simulink model "Target_Control_System"  (R2021b)
settings: Solver=FixedStepDiscrete  StartTime=0.0  StopTime=5  RelTol=1e-3
PreLoadFcn:
  | RTWConfigurationCB('preloadfcn', bdroot);
PostLoadFcn:
  | load('configuration/data_struct.mat');
  | load('configuration/fluxMaps_propMotor.mat');
  | load('configuration/parameterInit_PROP.mat');
  | load('configuration/parameterInit_PUMP.mat');
  | load('configuration/parameterInit_PITCH.mat');
  | load('configuration/parameterInit_TILT.mat');
  | %load('configuration/base_workspace_signal_definition.mat');
  | %load('resolvedatastores_to_baseworkspace_for_faster_simulation.mat');
model workspace (MAT data in the model file):
  SIMULATION_OPTIONS : Simulink.Parameter (value not decoded)
  TARGET_CODE_GEN : Simulink.Parameter (value not decoded)
  TCS_SAMPLE_FREQ_HZ : Simulink.Parameter (value not decoded)
symbols that are objects in the model workspace (value not decoded): TARGET_CODE_GEN, TCS_SAMPLE_FREQ_HZ
undefined symbols (not defined in the file): A_DQ_REF_LPF_INIT__PITCH, A_DQ_REF_LPF_INIT__PROP, A_DQ_REF_LPF_INIT__PUMP, A_DQ_REF_LPF_INIT__TILT, A_OBSERVER_CONFIDENCE_INIT__PITCH, A_OBSERVER_CONFIDENCE_INIT__PROP, A_OBSERVER_CONFIDENCE_INIT__PUMP, A_OBSERVER_CONFIDENCE_INIT__TILT, ACTUATOR_MAX_ANGLE_TRIP__PITCH, ACTUATOR_MIN_ANGLE_TRIP__PITCH, ACTUATOR_POS_SENSOR_INV_DIRECTION__PITCH, ACTUATOR_POS_SENSOR_INV_DIRECTION__TILT, ACTUATOR_POS_SENSOR_OFFSET__PITCH, ACTUATOR_POS_SENSOR_OFFSET__TILT, ADC_scaler1_baseaddr_TILT, ADC_SCALER_FLOAT_TO_FIXPOINT_EXPANSION, ANGLE_ELEC_FROM_SENSOR_OFFSET_INIT__PITCH, ANGLE_ELEC_FROM_SENSOR_OFFSET_INIT__PROP, ANGLE_ELEC_FROM_SENSOR_OFFSET_INIT__PUMP, ANGLE_ELEC_FROM_SENSOR_OFFSET_INIT__TILT, AUTO_CLEAR_FAULTS_ENABLED__PITCH, AUTO_CLEAR_FAULTS_ENABLED__PROP, AUTO_CLEAR_FAULTS_ENABLED__PUMP, AUTO_CLEAR_FAULTS_ENABLED__TILT, AUTO_CLEAR_FAULTS_WAIT_TICKS__PITCH, AUTO_CLEAR_FAULTS_WAIT_TICKS__PROP, AUTO_CLEAR_FAULTS_WAIT_TICKS__PUMP, AUTO_CLEAR_FAULTS_WAIT_TICKS__TILT, AUTO_I_ZERO_IDLE_TICKS__PITCH, AUTO_I_ZERO_IDLE_TICKS__PROP, AUTO_I_ZERO_IDLE_TICKS__PUMP, AUTO_I_ZERO_IDLE_TICKS__TILT, AUTO_I_ZERO_OFFSET_IDC_THRESHOLD__PITCH, AUTO_I_ZERO_OFFSET_IDC_THRESHOLD__PROP, AUTO_I_ZERO_OFFSET_IDC_THRESHOLD__PUMP, AUTO_I_ZERO_OFFSET_IDC_THRESHOLD__TILT, AUTO_I_ZERO_OFFSET_IPH_THRESHOLD__PITCH, AUTO_I_ZERO_OFFSET_IPH_THRESHOLD__PROP, AUTO_I_ZERO_OFFSET_IPH_THRESHOLD__PUMP, AUTO_I_ZERO_OFFSET_IPH_THRESHOLD__TILT, AUTO_SENSORLESS_SWITCHOVER_DISABLE_OMEGA, AUTO_SENSORLESS_SWITCHOVER_ENABLE_OMEGA, AUTO_SENSORLESS_SWITCHOVER_MIN_CONFIDENCE, AUXILIARY_PROTECTION_UNIT_BASEADDR__TILT, blanking_max_error_omega_INIT_PITCH, blanking_max_error_omega_INIT_TILT, blanking_max_error_position_INIT_PITCH, blanking_max_error_position_INIT_TILT, BRUTE_START_I_Q_REF_RAMP_SPEED__PITCH, BRUTE_START_I_Q_REF_RAMP_SPEED__PROP, BRUTE_START_I_Q_REF_RAMP_SPEED__PUMP, BRUTE_START_I_Q_REF_RAMP_SPEED__TILT, CONTROL_LOOP_DT_INIT__PITCH, CONTROL_LOOP_DT_INIT__PROP, CONTROL_LOOP_DT_INIT__PUMP, CONTROL_LOOP_DT_INIT__TILT, CORRECTION_FILTER_SCALE__PITCH, CORRECTION_FILTER_SCALE__PROP, CORRECTION_FILTER_SCALE__PUMP, CORRECTION_FILTER_SCALE__TILT ... (+458)
libraries: simulink x178, Reusables_Lib x24
(part 20 of 47)

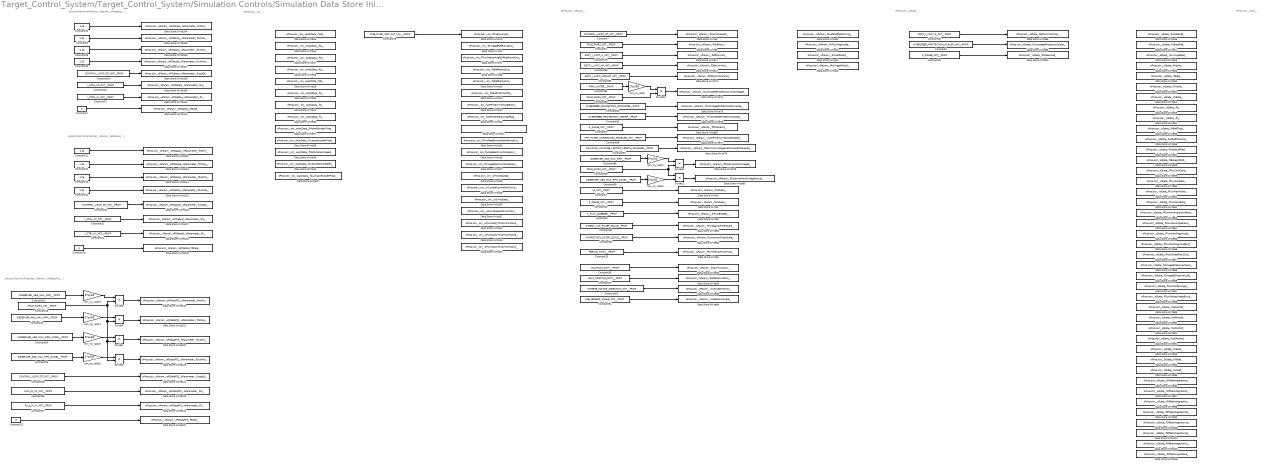
== system Target_Control_System/Target_Control_System/Simulation Controls/Simulation Data Store Initialization/parameter_init_prop/initializeIntTaskParametersPropulsion() ==
  note: oProp.oIsr_.oOut_...
  note: piControllerInit(oProp.oIsr_.oParam_.oPiDataPll2_...)
  note: piControllerInit(oProp.oIsr_.oParam_.oPiDataId_...)
  note: piControllerInit(oProp.oIsr_.oParam_.oPiDataIq_...)
  note: oProp.oIsr_.oState_...
  note: oProp.oIsr_.oIn_...
  note: oProp.oIsr_.oParam_...
  Constant1 : Constant  Value=0  OutDataTypeStr=single  SampleTime=-1
  Constant{10..11,13,29} (4 alike) : Constant  Value=-1.15  OutDataTypeStr=single  SampleTime=-1
  Constant{8,12,14,30} (4 alike) : Constant  Value=1.15  OutDataTypeStr=single  SampleTime=-1
  Constant15 : Constant  Value=0  OutDataTypeStr=single  SampleTime=-1
  Constant18 : Constant  Value=-OBSERVER_ABS_MAX_RPM__PROP  OutDataTypeStr=single  SampleTime=-1
  Constant{3,19,83,90} (4 alike) : Constant  Value=POLE_PAIRS_INIT__PROP  OutDataTypeStr=single  SampleTime=-1
  Constant2 : Constant  Value=LS_INIT__PROP  OutDataTypeStr=single  SampleTime=-1
  Constant20 : Constant  Value=OBSERVER_ABS_MAX_RPM__PROP  OutDataTypeStr=single  SampleTime=-1
  Constant21 : Constant  Value=I_CTRL_KI_INIT__PROP  OutDataTypeStr=single  SampleTime=-1
  Constant22 : Constant  Value=I_CTRL_KI_INIT__PROP  OutDataTypeStr=single  SampleTime=-1
  Constant23 : Constant  Value=0  OutDataTypeStr=single  SampleTime=-1
  Constant24 : Constant  Value=-OBSERVER_ABS_MAX_RPM_ACCEL__PROP  OutDataTypeStr=single  SampleTime=-1
  Constant25 : Constant  Value=PERIOD_TICKS__PROP  OutDataTypeStr=single  SampleTime=-1
  Constant26 : Constant  Value=OBSERVER_ABS_MAX_RPM_ACCEL__PROP  OutDataTypeStr=single  SampleTime=-1
  Constant27 : Constant  Value=PLL2_PI_KI_INIT__PROP  OutDataTypeStr=single  SampleTime=-1
  Constant{7,28,31,33} (4 alike) : Constant  Value=CONTROL_LOOP_DT_INIT__PROP  OutDataTypeStr=single  SampleTime=-1
  Constant32 : Constant  Value=I_CTRL_KP_INIT__PROP  OutDataTypeStr=single  SampleTime=-1
  Constant34 : Constant  Value=I_CTRL_KP_INIT__PROP  OutDataTypeStr=single  SampleTime=-1
  Constant35 : Constant  Value=PLL2_PI_KP_INIT__PROP  OutDataTypeStr=single  SampleTime=-1
  Constant37 : Constant  Value=HALF_POSITIVE_DUTY__PROP  OutDataTypeStr=single  SampleTime=-1
  Constant38 : Constant  Value=MAXIMUM_DUTY__PROP  OutDataTypeStr=single  SampleTime=-1
  Constant39 : Constant  Value=R_PHASE_INIT__PROP  OutDataTypeStr=single  SampleTime=-1
  Constant40 : Constant  Value=R_PHASE_INIT__PROP  OutDataTypeStr=single  SampleTime=-1
  Constant5 : Constant  Value=OVERSPEED_PROTECTION_SCALER_INIT__PROP  OutDataTypeStr=single  SampleTime=-1
  Constant6 : Constant  Value=R_PHASE_INIT__PROP  OutDataTypeStr=single  SampleTime=-1
  Constant78 : Constant  Value=ONE_OVER_UDC_INIT_VAL__PROP  OutDataTypeStr=single  SampleTime=-1
  Constant79 : Constant  Value=SOFT_I_LIMIT_A_INIT__PROP  OutDataTypeStr=single  SampleTime=-1
  Constant80 : Constant  Value=SOFT_I_LIMIT_KP_INIT__PROP  OutDataTypeStr=single  SampleTime=-1
  Constant81 : Constant  Value=SOFT_I_LIMIT_UPRAMP_INIT__PROP  OutDataTypeStr=single  SampleTime=-1
  Constant82 : Constant  Value=RPM_LIMITER__PROP  OutDataTypeStr=single  SampleTime=-1
  Constant84 : Constant  Value=OVERSPEED_PROTECTION_DOWNSTEP__PROP  OutDataTypeStr=single  SampleTime=-1
  Constant85 : Constant  Value=OVERSPEED_PROTECTION_UPSTEP__PROP  OutDataTypeStr=single  SampleTime=-1
  Constant86 : Constant  Value=UPH_FILTER_CORRECTION_ENABLED_INIT__PROP  OutDataTypeStr=uint32  SampleTime=-1
  Constant87 : Constant  Value=MAXIMUM_VOLTAGE_VECTOR_LENGTH_SQUARED__PROP  OutDataTypeStr=single  SampleTime=-1
  Constant88 : Constant  Value=OBSERVER_ABS_MAX_RPM__PROP  OutDataTypeStr=single  SampleTime=-1
  Constant89 : Constant  Value=OBSERVER_ABS_MAX_RPM_ACCEL__PROP  OutDataTypeStr=single  SampleTime=-1
  Constant9 : Constant  Value=K_FLUX_BLEEDER__PROP  OutDataTypeStr=single  SampleTime=-1
  Constant91 : Constant  Value=OMEGA_VAR_FILTER_SCALE__PROP  OutDataTypeStr=single  SampleTime=-1
  Constant92 : Constant  Value=CORRECTION_FILTER_SCALE__PROP  OutDataTypeStr=single  SampleTime=-1
  Constant93 : Constant  Value=INVERSE_MOTOR_DIRECTION_INIT__PROP  OutDataTypeStr=int32  SampleTime=-1
  Constant94 : Constant  Value=USE_SENSOR_ANGLE_INIT__PROP  OutDataTypeStr=int32  SampleTime=-1
  Constant95 : Constant  Value=SOFT_I_LIMIT_A_INIT__PROP  OutDataTypeStr=single  SampleTime=-1
  Data Store Write1 : DataStoreWrite  DataStoreName=oProp  DataStoreElements=oProp.oIsr_.oIn_.fOmegaERefRampOut_  IndexOptions=Index vector (dialog)  Indices=1  OutputSizes=1
  Data Store Write10 : DataStoreWrite  DataStoreName=oProp  DataStoreElements=oProp.oIsr_.oIn_.fIdRefRampOut_  IndexOptions=Index vector (dialog)  Indices=1  OutputSizes=1
  Data Store Write100 : DataStoreWrite  DataStoreName=oProp  DataStoreElements=oProp.oIsr_.oState_.fOffsetIntegratorUa_  IndexOptions=Index vector (dialog)  Indices=1  OutputSizes=1
  Data Store Write101 : DataStoreWrite  DataStoreName=oProp  DataStoreElements=oProp.oIsr_.oState_.fOffsetIntegratorUb_  IndexOptions=Index vector (dialog)  Indices=1  OutputSizes=1
  Data Store Write102 : DataStoreWrite  DataStoreName=oProp  DataStoreElements=oProp.oIsr_.oState_.fOffsetIntegratorUc_  IndexOptions=Index vector (dialog)  Indices=1  OutputSizes=1
  Data Store Write103 : DataStoreWrite  DataStoreName=oProp  DataStoreElements=oProp.oIsr_.oState_.fOffsetAvgUphase_  IndexOptions=Index vector (dialog)  Indices=1  OutputSizes=1
  Data Store Write104 : DataStoreWrite  DataStoreName=oProp  DataStoreElements=oProp.oIsr_.oParam_.oPiDataIq_.oParameter_.fIntMin_  IndexOptions=Index vector (dialog)  Indices=1  OutputSizes=1
  Data Store Write105 : DataStoreWrite  DataStoreName=oProp  DataStoreElements=oProp.oIsr_.oParam_.oPiDataIq_.oParameter_.fIntMax_  IndexOptions=Index vector (dialog)  Indices=1  OutputSizes=1
  Data Store Write106 : DataStoreWrite  DataStoreName=oProp  DataStoreElements=oProp.oIsr_.oParam_.oPiDataIq_.oParameter_.fOutMin_  IndexOptions=Index vector (dialog)  Indices=1  OutputSizes=1
  Data Store Write107 : DataStoreWrite  DataStoreName=oProp  DataStoreElements=oProp.oIsr_.oParam_.oPiDataIq_.oParameter_.fOutMax_  IndexOptions=Index vector (dialog)  Indices=1  OutputSizes=1
  Data Store Write108 : DataStoreWrite  DataStoreName=oProp  DataStoreElements=oProp.oIsr_.oParam_.oPiDataIq_.oParameter_.fLoopDt_  IndexOptions=Index vector (dialog)  Indices=1  OutputSizes=1
  Data Store Write109 : DataStoreWrite  DataStoreName=oProp  DataStoreElements=oProp.oIsr_.oParam_.oPiDataIq_.oParameter_.fKp_  IndexOptions=Index vector (dialog)  Indices=1  OutputSizes=1
  Data Store Write11 : DataStoreWrite  DataStoreName=oProp  DataStoreElements=oProp.oIsr_.oIn_.fIdRefFractionOfIq_  IndexOptions=Index vector (dialog)  Indices=1  OutputSizes=1
  Data Store Write110 : DataStoreWrite  DataStoreName=oProp  DataStoreElements=oProp.oIsr_.oParam_.oPiDataIq_.oParameter_.fKi_  IndexOptions=Index vector (dialog)  Indices=1  OutputSizes=1
  Data Store Write111 : DataStoreWrite  DataStoreName=oProp  DataStoreElements=oProp.oIsr_.oParam_.oPiDataIq_.fState_  IndexOptions=Index vector (dialog)  Indices=1  OutputSizes=1
  Data Store Write112 : DataStoreWrite  DataStoreName=oProp  DataStoreElements=oProp.oIsr_.oParam_.oPiDataId_.oParameter_.fIntMin_  IndexOptions=Index vector (dialog)  Indices=1  OutputSizes=1
  Data Store Write113 : DataStoreWrite  DataStoreName=oProp  DataStoreElements=oProp.oIsr_.oParam_.oPiDataId_.oParameter_.fIntMax_  IndexOptions=Index vector (dialog)  Indices=1  OutputSizes=1
  Data Store Write114 : DataStoreWrite  DataStoreName=oProp  DataStoreElements=oProp.oIsr_.oParam_.oPiDataId_.oParameter_.fOutMin_  IndexOptions=Index vector (dialog)  Indices=1  OutputSizes=1
  Data Store Write115 : DataStoreWrite  DataStoreName=oProp  DataStoreElements=oProp.oIsr_.oParam_.oPiDataId_.oParameter_.fOutMax_  IndexOptions=Index vector (dialog)  Indices=1  OutputSizes=1
  Data Store Write116 : DataStoreWrite  DataStoreName=oProp  DataStoreElements=oProp.oIsr_.oParam_.oPiDataId_.oParameter_.fLoopDt_  IndexOptions=Index vector (dialog)  Indices=1  OutputSizes=1
  Data Store Write117 : DataStoreWrite  DataStoreName=oProp  DataStoreElements=oProp.oIsr_.oParam_.oPiDataId_.oParameter_.fKp_  IndexOptions=Index vector (dialog)  Indices=1  OutputSizes=1
  Data Store Write118 : DataStoreWrite  DataStoreName=oProp  DataStoreElements=oProp.oIsr_.oParam_.oPiDataId_.oParameter_.fKi_  IndexOptions=Index vector (dialog)  Indices=1  OutputSizes=1
  Data Store Write119 : DataStoreWrite  DataStoreName=oProp  DataStoreElements=oProp.oIsr_.oParam_.oPiDataId_.fState_  IndexOptions=Index vector (dialog)  Indices=1  OutputSizes=1
  Data Store Write12 : DataStoreWrite  DataStoreName=oProp  DataStoreElements=oProp.oIsr_.oIn_.fUphFilterAmplitudeRatio_  IndexOptions=Index vector (dialog)  Indices=1  OutputSizes=1
  Data Store Write120 : DataStoreWrite  DataStoreName=oProp  DataStoreElements=oProp.oIsr_.oParam_.oPiDataPll2_.oParameter_.fIntMin_  IndexOptions=Index vector (dialog)  Indices=1  OutputSizes=1
  Data Store Write121 : DataStoreWrite  DataStoreName=oProp  DataStoreElements=oProp.oIsr_.oParam_.oPiDataPll2_.oParameter_.fIntMax_  IndexOptions=Index vector (dialog)  Indices=1  OutputSizes=1
  Data Store Write122 : DataStoreWrite  DataStoreName=oProp  DataStoreElements=oProp.oIsr_.oParam_.oPiDataPll2_.oParameter_.fOutMin_  IndexOptions=Index vector (dialog)  Indices=1  OutputSizes=1
  Data Store Write123 : DataStoreWrite  DataStoreName=oProp  DataStoreElements=oProp.oIsr_.oParam_.oPiDataPll2_.oParameter_.fOutMax_  IndexOptions=Index vector (dialog)  Indices=1  OutputSizes=1
  Data Store Write124 : DataStoreWrite  DataStoreName=oProp  DataStoreElements=oProp.oIsr_.oParam_.oPiDataPll2_.oParameter_.fLoopDt_  IndexOptions=Index vector (dialog)  Indices=1  OutputSizes=1
  Data Store Write125 : DataStoreWrite  DataStoreName=oProp  DataStoreElements=oProp.oIsr_.oParam_.oPiDataPll2_.oParameter_.fKi_  IndexOptions=Index vector (dialog)  Indices=1  OutputSizes=1
  Data Store Write126 : DataStoreWrite  DataStoreName=oProp  DataStoreElements=oProp.oIsr_.oParam_.oPiDataPll2_.oParameter_.fKp_  IndexOptions=Index vector (dialog)  Indices=1  OutputSizes=1
  Data Store Write127 : DataStoreWrite  DataStoreName=oProp  DataStoreElements=oProp.oIsr_.oParam_.oPiDataPll2_.fState_  IndexOptions=Index vector (dialog)  Indices=1  OutputSizes=1
  Data Store Write13 : DataStoreWrite  DataStoreName=oProp  DataStoreElements=oProp.oIsr_.oIn_.fUphFilterDelayAngleRad_  IndexOptions=Index vector (dialog)  Indices=1  OutputSizes=1
  Data Store Write14 : DataStoreWrite  DataStoreName=oProp  DataStoreElements=oProp.oIsr_.oIn_.fFluxMasterAngleForced2closedSmoothingRampOut_  IndexOptions=Index vector (dialog)  Indices=1  OutputSizes=1
  Data Store Write15 : DataStoreWrite  DataStoreName=oProp  DataStoreElements=oProp.oIsr_.oIn_.fFluxFeedforwardGainRampOut_  IndexOptions=Index vector (dialog)  Indices=1  OutputSizes=1
  Data Store Write16 : DataStoreWrite  DataStoreName=oProp  DataStoreElements=oProp.oIsr_.oIn_.fAngleElecFromPosSensor_  IndexOptions=Index vector (dialog)  Indices=1  OutputSizes=1
  Data Store Write17 : DataStoreWrite  DataStoreName=oProp  DataStoreElements=oProp.oIsr_.oIn_.fOmegaElecFromPosSensor_  IndexOptions=Index vector (dialog)  Indices=1  OutputSizes=1
  Data Store Write18 : DataStoreWrite  DataStoreName=oProp  DataStoreElements=oProp.oIsr_.oIn_.uiForcedAngle_  IndexOptions=Index vector (dialog)  Indices=1  OutputSizes=1
  Data Store Write19 : DataStoreWrite  DataStoreName=oProp  DataStoreElements=oProp.oIsr_.oIn_.uiCurrentControllerActive_  IndexOptions=Index vector (dialog)  Indices=1  OutputSizes=1
  Data Store Write2 : DataStoreWrite  DataStoreName=oProp  DataStoreElements=oProp.oIsr_.oParam_.fRsPhase_  IndexOptions=Index vector (dialog)  Indices=1  OutputSizes=1
  Data Store Write20 : DataStoreWrite  DataStoreName=oProp  DataStoreElements=oProp.oIsr_.oIn_.uiDriveState_  IndexOptions=Index vector (dialog)  Indices=1  OutputSizes=1
  Data Store Write21 : DataStoreWrite  DataStoreName=oProp  DataStoreElements=oProp.oIsr_.oIn_.uiPwmRequestFromMain_  IndexOptions=Index vector (dialog)  Indices=1  OutputSizes=1
  Data Store Write22 : DataStoreWrite  DataStoreName=oProp  DataStoreElements=oProp.oIsr_.oIn_.uiPwmDutyTicksFromMainA_  IndexOptions=Index vector (dialog)  Indices=1  OutputSizes=1
  Data Store Write23 : DataStoreWrite  DataStoreName=oProp  DataStoreElements=oProp.oIsr_.oIn_.uiPwmDutyTicksFromMainB_  IndexOptions=Index vector (dialog)  Indices=1  OutputSizes=1
  Data Store Write24 : DataStoreWrite  DataStoreName=oProp  DataStoreElements=oProp.oIsr_.oIn_.uiPwmDutyTicksFromMainC_  IndexOptions=Index vector (dialog)  Indices=1  OutputSizes=1
  Data Store Write25 : DataStoreWrite  DataStoreName=oProp  DataStoreElements=oProp.oIsr_.oIn_.oAdcData_.fUdc_  IndexOptions=Index vector (dialog)  Indices=1  OutputSizes=1
  Data Store Write26 : DataStoreWrite  DataStoreName=oProp  DataStoreElements=oProp.oIsr_.oIn_.oAdcData_.fUa_  IndexOptions=Index vector (dialog)  Indices=1  OutputSizes=1
  Data Store Write27 : DataStoreWrite  DataStoreName=oProp  DataStoreElements=oProp.oIsr_.oIn_.oAdcData_.fUb_  IndexOptions=Index vector (dialog)  Indices=1  OutputSizes=1
  Data Store Write28 : DataStoreWrite  DataStoreName=oProp  DataStoreElements=oProp.oIsr_.oIn_.oAdcData_.fUc_  IndexOptions=Index vector (dialog)  Indices=1  OutputSizes=1
  Data Store Write29 : DataStoreWrite  DataStoreName=oProp  DataStoreElements=oProp.oIsr_.oIn_.oAdcData_.fIdc_  IndexOptions=Index vector (dialog)  Indices=1  OutputSizes=1
  Data Store Write3 : DataStoreWrite  DataStoreName=oProp  DataStoreElements=oProp.oIsr_.oParam_.fPolePairs_  IndexOptions=Index vector (dialog)  Indices=1  OutputSizes=1
  Data Store Write30 : DataStoreWrite  DataStoreName=oProp  DataStoreElements=oProp.oIsr_.oIn_.oAdcData_.fIa_  IndexOptions=Index vector (dialog)  Indices=1  OutputSizes=1
  Data Store Write31 : DataStoreWrite  DataStoreName=oProp  DataStoreElements=oProp.oIsr_.oIn_.oAdcData_.fIb_  IndexOptions=Index vector (dialog)  Indices=1  OutputSizes=1
  Data Store Write32 : DataStoreWrite  DataStoreName=oProp  DataStoreElements=oProp.oIsr_.oParam_.fMaximumDuty_  IndexOptions=Index vector (dialog)  Indices=1  OutputSizes=1
  Data Store Write33 : DataStoreWrite  DataStoreName=oProp  DataStoreElements=oProp.oIsr_.oParam_.fHalfPositiveDuty_  IndexOptions=Index vector (dialog)  Indices=1  OutputSizes=1
  Data Store Write34 : DataStoreWrite  DataStoreName=oProp  DataStoreElements=oProp.oIsr_.oState_.fRMeasured_  IndexOptions=Index vector (dialog)  Indices=1  OutputSizes=1
  Data Store Write35 : DataStoreWrite  DataStoreName=oProp  DataStoreElements=oProp.oIsr_.oParam_.fRPhaseInit_  IndexOptions=Index vector (dialog)  Indices=1  OutputSizes=1
  Data Store Write36 : DataStoreWrite  DataStoreName=oProp  DataStoreElements=oProp.oIsr_.oIn_.oAdcData_.fIc_  IndexOptions=Index vector (dialog)  Indices=1  OutputSizes=1
  Data Store Write37 : DataStoreWrite  DataStoreName=oProp  DataStoreElements=oProp.oIsr_.oIn_.oAdcData_.fMotorEncoderFloat_  IndexOptions=Index vector (dialog)  Indices=1  OutputSizes=1
  Data Store Write38 : DataStoreWrite  DataStoreName=oProp  DataStoreElements=oProp.oIsr_.oIn_.oAdcData_.fOutputEncoderFloat_  IndexOptions=Index vector (dialog)  Indices=1  OutputSizes=1
  Data Store Write39 : DataStoreWrite  DataStoreName=oProp  DataStoreElements=oProp.oIsr_.oIn_.oAdcData_.fMotorSensorSpeed_  IndexOptions=Index vector (dialog)  Indices=1  OutputSizes=1
  Data Store Write4 : DataStoreWrite  DataStoreName=oProp  DataStoreElements=oProp.oIsr_.oParam_.fLsPhase_  IndexOptions=Index vector (dialog)  Indices=1  OutputSizes=1
  Data Store Write40 : DataStoreWrite  DataStoreName=oProp  DataStoreElements=oProp.oIsr_.oIn_.oAdcData_.fOutputSensorSpeed_  IndexOptions=Index vector (dialog)  Indices=1  OutputSizes=1
  Data Store Write41 : DataStoreWrite  DataStoreName=oProp  DataStoreElements=oProp.oIsr_.oIn_.oAdcData_.fAuxiliaryEncoderFloat_  IndexOptions=Index vector (dialog)  Indices=1  OutputSizes=1
  Data Store Write42 : DataStoreWrite  DataStoreName=oProp  DataStoreElements=oProp.oIsr_.oParam_.fALpf4hpfDcBlocking_  IndexOptions=Index vector (dialog)  Indices=1  OutputSizes=1
  Data Store Write43 : DataStoreWrite  DataStoreName=oProp  DataStoreElements=oProp.oIsr_.oParam_.fAFluxMagnitude_  IndexOptions=Index vector (dialog)  Indices=1  OutputSizes=1
  Data Store Write44 : DataStoreWrite  DataStoreName=oProp  DataStoreElements=oProp.oIsr_.oParam_.fALoopfilter2_  IndexOptions=Index vector (dialog)  Indices=1  OutputSizes=1
  Data Store Write45 : DataStoreWrite  DataStoreName=oProp  DataStoreElements=oProp.oIsr_.oParam_.fAOmegaFilter2_  IndexOptions=Index vector (dialog)  Indices=1  OutputSizes=1
  Data Store Write46 : DataStoreWrite  DataStoreName=oProp  DataStoreElements=oProp.oIsr_.oState_.fUAlphaRef_  IndexOptions=Index vector (dialog)  Indices=1  OutputSizes=1
  Data Store Write47 : DataStoreWrite  DataStoreName=oProp  DataStoreElements=oProp.oIsr_.oState_.fUBetaRef_  IndexOptions=Index vector (dialog)  Indices=1  OutputSizes=1
  Data Store Write48 : DataStoreWrite  DataStoreName=oProp  DataStoreElements=oProp.oIsr_.oState_.iPwmUpdated_  IndexOptions=Index vector (dialog)  Indices=1  OutputSizes=1
  Data Store Write49 : DataStoreWrite  DataStoreName=oProp  DataStoreElements=oProp.oIsr_.oState_.fIAlpha_  IndexOptions=Index vector (dialog)  Indices=1  OutputSizes=1
  Data Store Write5 : DataStoreWrite  DataStoreName=oProp  DataStoreElements=oProp.oIsr_.oParam_.fControlLoopDt_  IndexOptions=Index vector (dialog)  Indices=1  OutputSizes=1
  Data Store Write50 : DataStoreWrite  DataStoreName=oProp  DataStoreElements=oProp.oIsr_.oState_.fIBeta_  IndexOptions=Index vector (dialog)  Indices=1  OutputSizes=1
  Data Store Write51 : DataStoreWrite  DataStoreName=oProp  DataStoreElements=oProp.oIsr_.oState_.fUAlpha_  IndexOptions=Index vector (dialog)  Indices=1  OutputSizes=1
  Data Store Write52 : DataStoreWrite  DataStoreName=oProp  DataStoreElements=oProp.oIsr_.oState_.fUBeta_  IndexOptions=Index vector (dialog)  Indices=1  OutputSizes=1
  Data Store Write53 : DataStoreWrite  DataStoreName=oProp  DataStoreElements=oProp.oIsr_.oState_.fId_  IndexOptions=Index vector (dialog)  Indices=1  OutputSizes=1
  Data Store Write54 : DataStoreWrite  DataStoreName=oProp  DataStoreElements=oProp.oIsr_.oState_.fIq_  IndexOptions=Index vector (dialog)  Indices=1  OutputSizes=1
  Data Store Write55 : DataStoreWrite  DataStoreName=oProp  DataStoreElements=oProp.oIsr_.oState_.fIdRefTotal_  IndexOptions=Index vector (dialog)  Indices=1  OutputSizes=1
  Data Store Write56 : DataStoreWrite  DataStoreName=oProp  DataStoreElements=oProp.oIsr_.oState_.fUqRefPiContrib_  IndexOptions=Index vector (dialog)  Indices=1  OutputSizes=1
  Data Store Write57 : DataStoreWrite  DataStoreName=oProp  DataStoreElements=oProp.oIsr_.oState_.fIAlphaLpf4hpf_  IndexOptions=Index vector (dialog)  Indices=1  OutputSizes=1
  Data Store Write58 : DataStoreWrite  DataStoreName=oProp  DataStoreElements=oProp.oIsr_.oState_.fIBetaLpf4hpf_  IndexOptions=Index vector (dialog)  Indices=1  OutputSizes=1
  Data Store Write59 : DataStoreWrite  DataStoreName=oProp  DataStoreElements=oProp.oIsr_.oState_.fFluxCoilAlpha_  IndexOptions=Index vector (dialog)  Indices=1  OutputSizes=1
  Data Store Write6 : DataStoreWrite  DataStoreName=oProp  DataStoreElements=oProp.oIsr_.oParam_.fKFluxBleeder_  IndexOptions=Index vector (dialog)  Indices=1  OutputSizes=1
  Data Store Write60 : DataStoreWrite  DataStoreName=oProp  DataStoreElements=oProp.oIsr_.oState_.fFluxCoilBeta_  IndexOptions=Index vector (dialog)  Indices=1  OutputSizes=1
  Data Store Write61 : DataStoreWrite  DataStoreName=oProp  DataStoreElements=oProp.oIsr_.oState_.fFluxMainAlpha_  IndexOptions=Index vector (dialog)  Indices=1  OutputSizes=1
  Data Store Write62 : DataStoreWrite  DataStoreName=oProp  DataStoreElements=oProp.oIsr_.oState_.fFluxMainBeta_  IndexOptions=Index vector (dialog)  Indices=1  OutputSizes=1
  Data Store Write63 : DataStoreWrite  DataStoreName=oProp  DataStoreElements=oProp.oIsr_.oState_.fFluxMainAngleUltraRaw_  IndexOptions=Index vector (dialog)  Indices=1  OutputSizes=1
  Data Store Write64 : DataStoreWrite  DataStoreName=oProp  DataStoreElements=oProp.oIsr_.oState_.fFluxMainAngleRaw2_  IndexOptions=Index vector (dialog)  Indices=1  OutputSizes=1
  Data Store Write65 : DataStoreWrite  DataStoreName=oProp  DataStoreElements=oProp.oIsr_.oState_.fFluxMainMagnitude_  IndexOptions=Index vector (dialog)  Indices=1  OutputSizes=1
  Data Store Write66 : DataStoreWrite  DataStoreName=oProp  DataStoreElements=oProp.oIsr_.oState_.fFluxMainMagnitudeLpf_  IndexOptions=Index vector (dialog)  Indices=1  OutputSizes=1
  Data Store Write67 : DataStoreWrite  DataStoreName=oProp  DataStoreElements=oProp.oIsr_.oState_.fAtan2loopfilter2Out_  IndexOptions=Index vector (dialog)  Indices=1  OutputSizes=1
  Data Store Write68 : DataStoreWrite  DataStoreName=oProp  DataStoreElements=oProp.oIsr_.oState_.fOmegaEObserverRaw2_  IndexOptions=Index vector (dialog)  Indices=1  OutputSizes=1
  Data Store Write69 : DataStoreWrite  DataStoreName=oProp  DataStoreElements=oProp.oIsr_.oState_.fOmegaEObserverLpf2_  IndexOptions=Index vector (dialog)  Indices=1  OutputSizes=1
  Data Store Write7 : DataStoreWrite  DataStoreName=oProp  DataStoreElements=oProp.oIsr_.oIn_.fFluxMasterAngleOffsetRampOut_  IndexOptions=Index vector (dialog)  Indices=1  OutputSizes=1
  Data Store Write70 : DataStoreWrite  DataStoreName=oProp  DataStoreElements=oProp.oIsr_.oIn_.fOneOverUdc_  IndexOptions=Index vector (dialog)  Indices=1  OutputSizes=1
  Data Store Write71 : DataStoreWrite  DataStoreName=oProp  DataStoreElements=oProp.oIsr_.oParam_.fSoftILimitA_  IndexOptions=Index vector (dialog)  Indices=1  OutputSizes=1
  Data Store Write72 : DataStoreWrite  DataStoreName=oProp  DataStoreElements=oProp.oIsr_.oParam_.fSoftILimitKp_  IndexOptions=Index vector (dialog)  Indices=1  OutputSizes=1
  Data Store Write73 : DataStoreWrite  DataStoreName=oProp  DataStoreElements=oProp.oIsr_.oParam_.fSoftILimitUpramp_  IndexOptions=Index vector (dialog)  Indices=1  OutputSizes=1
  Data Store Write74 : DataStoreWrite  DataStoreName=oProp  DataStoreElements=oProp.oIsr_.oParam_.fOverspeedProtectionLimitOmegaE_  IndexOptions=Index vector (dialog)  Indices=1  OutputSizes=1
  Data Store Write75 : DataStoreWrite  DataStoreName=oProp  DataStoreElements=oProp.oIsr_.oParam_.fOverspeedProtectionDownstep_  IndexOptions=Index vector (dialog)  Indices=1  OutputSizes=1
  Data Store Write76 : DataStoreWrite  DataStoreName=oProp  DataStoreElements=oProp.oIsr_.oParam_.fOverspeedProtectionUpstep_  IndexOptions=Index vector (dialog)  Indices=1  OutputSizes=1
  Data Store Write77 : DataStoreWrite  DataStoreName=oProp  DataStoreElements=oProp.oIsr_.oParam_.uiUphFilterCorrectionEnabled_  IndexOptions=Index vector (dialog)  Indices=1  OutputSizes=1
  Data Store Write78 : DataStoreWrite  DataStoreName=oProp  DataStoreElements=oProp.oIsr_.oParam_.fMaximumVoltageVectorLengthSquared_  IndexOptions=Index vector (dialog)  Indices=1  OutputSizes=1
  Data Store Write79 : DataStoreWrite  DataStoreName=oProp  DataStoreElements=oProp.oIsr_.oParam_.fObserverMaxOmegaE_  IndexOptions=Index vector (dialog)  Indices=1  OutputSizes=1
  Data Store Write8 : DataStoreWrite  DataStoreName=oProp  DataStoreElements=oProp.oIsr_.oIn_.fIqRefRampOut_  IndexOptions=Index vector (dialog)  Indices=1  OutputSizes=1
  Data Store Write80 : DataStoreWrite  DataStoreName=oProp  DataStoreElements=oProp.oIsr_.oParam_.fObserverMaxOmegaEAccel_  IndexOptions=Index vector (dialog)  Indices=1  OutputSizes=1
  Data Store Write81 : DataStoreWrite  DataStoreName=oProp  DataStoreElements=oProp.oIsr_.oParam_.fOmegaVarFilterScale_  IndexOptions=Index vector (dialog)  Indices=1  OutputSizes=1
  Data Store Write82 : DataStoreWrite  DataStoreName=oProp  DataStoreElements=oProp.oIsr_.oParam_.fCorrectionFilterScale_  IndexOptions=Index vector (dialog)  Indices=1  OutputSizes=1
  Data Store Write83 : DataStoreWrite  DataStoreName=oProp  DataStoreElements=oProp.oIsr_.oParam_.iInverseDirection_  IndexOptions=Index vector (dialog)  Indices=1  OutputSizes=1
  Data Store Write84 : DataStoreWrite  DataStoreName=oProp  DataStoreElements=oProp.oIsr_.oParam_.iUseSensorAngle_  IndexOptions=Index vector (dialog)  Indices=1  OutputSizes=1
  Data Store Write85 : DataStoreWrite  DataStoreName=oProp  DataStoreElements=oProp.oIsr_.oState_.fSoftILimitActual_  IndexOptions=Index vector (dialog)  Indices=1  OutputSizes=1
  Data Store Write86 : DataStoreWrite  DataStoreName=oProp  DataStoreElements=oProp.oIsr_.oState_.fOverspeedProtectionScaler_  IndexOptions=Index vector (dialog)  Indices=1  OutputSizes=1
  Data Store Write87 : DataStoreWrite  DataStoreName=oProp  DataStoreElements=oProp.oIsr_.oState_.fFluxMasterAngle_  IndexOptions=Index vector (dialog)  Indices=1  OutputSizes=1
  Data Store Write88 : DataStoreWrite  DataStoreName=oProp  DataStoreElements=oProp.oIsr_.oState_.fFluxMasterAngleBkwd_  IndexOptions=Index vector (dialog)  Indices=1  OutputSizes=1
  Data Store Write89 : DataStoreWrite  DataStoreName=oProp  DataStoreElements=oProp.oIsr_.oState_.fUaPostlpf_  IndexOptions=Index vector (dialog)  Indices=1  OutputSizes=1
  Data Store Write9 : DataStoreWrite  DataStoreName=oProp  DataStoreElements=oProp.oIsr_.oParam_.fPwmPeriodTicksFloat_  IndexOptions=Index vector (dialog)  Indices=1  OutputSizes=1
  Data Store Write90 : DataStoreWrite  DataStoreName=oProp  DataStoreElements=oProp.oIsr_.oState_.fUbPostlpf_  IndexOptions=Index vector (dialog)  Indices=1  OutputSizes=1
  Data Store Write91 : DataStoreWrite  DataStoreName=oProp  DataStoreElements=oProp.oIsr_.oState_.fUcPostlpf_  IndexOptions=Index vector (dialog)  Indices=1  OutputSizes=1
  Data Store Write92 : DataStoreWrite  DataStoreName=oProp  DataStoreElements=oProp.oIsr_.oState_.fUdcPostlpf_  IndexOptions=Index vector (dialog)  Indices=1  OutputSizes=1
  Data Store Write93 : DataStoreWrite  DataStoreName=oProp  DataStoreElements=oProp.oIsr_.oState_.fUaRef_  IndexOptions=Index vector (dialog)  Indices=1  OutputSizes=1
  Data Store Write94 : DataStoreWrite  DataStoreName=oProp  DataStoreElements=oProp.oIsr_.oState_.fUbRef_  IndexOptions=Index vector (dialog)  Indices=1  OutputSizes=1
  Data Store Write95 : DataStoreWrite  DataStoreName=oProp  DataStoreElements=oProp.oIsr_.oState_.fUcRef_  IndexOptions=Index vector (dialog)  Indices=1  OutputSizes=1
  Data Store Write96 : DataStoreWrite  DataStoreName=oProp  DataStoreElements=oProp.oIsr_.oState_.fOffsetIntegratorIa_  IndexOptions=Index vector (dialog)  Indices=1  OutputSizes=1
  Data Store Write97 : DataStoreWrite  DataStoreName=oProp  DataStoreElements=oProp.oIsr_.oState_.fOffsetIntegratorIb_  IndexOptions=Index vector (dialog)  Indices=1  OutputSizes=1
  Data Store Write98 : DataStoreWrite  DataStoreName=oProp  DataStoreElements=oProp.oIsr_.oState_.fOffsetIntegratorIc_  IndexOptions=Index vector (dialog)  Indices=1  OutputSizes=1
  Data Store Write99 : DataStoreWrite  DataStoreName=oProp  DataStoreElements=oProp.oIsr_.oState_.fOffsetIntegratorIdc_  IndexOptions=Index vector (dialog)  Indices=1  OutputSizes=1
  Divide{1,3..5} (4 alike) : Product  Inputs=**  OutDataTypeStr=single
  Divide10 : Product  Inputs=**
  Divide11 : Product  Inputs=**
  Divide12 : Product  Inputs=**
  rpm_to_rad/s : Gain  Gain=2*pi/60
  rpm_to_rad/s1 : Gain  Gain=2*pi/60
  rpm_to_rad/s2 : Gain  Gain=2*pi/60
  rpm_to_rad/s{3..6} (4 alike) : Gain  Gain=2*pi/60  OutDataTypeStr=single
  wires:
  Constant35/1 -> Data Store Write126/1
  Constant27/1 -> Data Store Write125/1
  Constant25/1 -> Data Store Write9/1
  Constant23/1 -> Data Store Write127/1
  Divide5/1 -> Data Store Write123/1
  rpm_to_rad/s6/1 -> Divide5/1
  Divide1/1 -> Data Store Write122/1
  rpm_to_rad/s5/1 -> Divide1/1
  Divide4/1 -> Data Store Write121/1
  rpm_to_rad/s4/1 -> Divide4/1
  Constant24/1 -> rpm_to_rad/s5/1
  Constant20/1 -> rpm_to_rad/s4/1
  Divide3/1 -> Data Store Write120/1
  Constant19/1 -> Divide3/2, Divide4/2, Divide1/2, Divide5/2
  rpm_to_rad/s3/1 -> Divide3/1
  Constant18/1 -> rpm_to_rad/s3/1
  Constant26/1 -> rpm_to_rad/s6/1
  Constant28/1 -> Data Store Write124/1
  Constant15/1 -> Data Store Write119/1
  Constant14/1 -> Data Store Write115/1
  Constant13/1 -> Data Store Write114/1
  Constant21/1 -> Data Store Write118/1
  Constant12/1 -> Data Store Write113/1
  Constant31/1 -> Data Store Write116/1
  Constant11/1 -> Data Store Write112/1
  Constant32/1 -> Data Store Write117/1
  Constant1/1 -> Data Store Write111/1
  Constant33/1 -> Data Store Write108/1
  Constant34/1 -> Data Store Write109/1
  Constant30/1 -> Data Store Write107/1
  Constant22/1 -> Data Store Write110/1
  Constant29/1 -> Data Store Write106/1
  Constant10/1 -> Data Store Write104/1
  Constant8/1 -> Data Store Write105/1
  Constant80/1 -> Data Store Write72/1
  Constant5/1 -> Data Store Write86/1
  Constant92/1 -> Data Store Write82/1
  Divide11/1 -> Data Store Write79/1
  Divide12/1 -> Data Store Write80/1
  Constant85/1 -> Data Store Write76/1
  Constant6/1 -> Data Store Write35/1
  Constant82/1 -> rpm_to_rad/s/1
  Divide10/1 -> Data Store Write74/1
  Constant84/1 -> Data Store Write75/1
  rpm_to_rad/s2/1 -> Divide12/2
  Constant88/1 -> rpm_to_rad/s1/1
  Constant78/1 -> Data Store Write70/1
  rpm_to_rad/s/1 -> Divide10/1
  Constant93/1 -> Data Store Write83/1
  Constant86/1 -> Data Store Write77/1
  Constant95/1 -> Data Store Write85/1
  Constant2/1 -> Data Store Write4/1
  Constant87/1 -> Data Store Write78/1
  Constant3/1 -> Data Store Write3/1
  Constant40/1 -> Data Store Write2/1
  Constant90/1 -> Divide11/2, Divide12/1
  Constant91/1 -> Data Store Write81/1
  Constant39/1 -> Data Store Write34/1
  Constant79/1 -> Data Store Write71/1
  Constant94/1 -> Data Store Write84/1
  Constant83/1 -> Divide10/2
  Constant9/1 -> Data Store Write6/1
  Constant89/1 -> rpm_to_rad/s2/1
  Constant81/1 -> Data Store Write73/1
  Constant38/1 -> Data Store Write32/1
  rpm_to_rad/s1/1 -> Divide11/1
  Constant37/1 -> Data Store Write33/1
  Constant7/1 -> Data Store Write5/1
